simulink model "stateflow_test"  (R2021a)
settings: Solver=FixedStepAuto  StartTime=0.0  StopTime=10.0  FixedStep=1/64  RelTol=1e-3
settings Model: OrderedModelArguments=off  Creator=Jack-STK2  LastModifiedBy=jacky

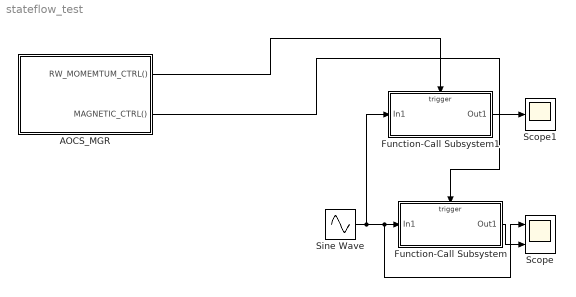
== system stateflow_test ==
  AOCS_MGR : Stateflow chart  TreatAsAtomicUnit=on  SystemSampleTime=1/8
  Function-Call Subsystem : Subsystem  TreatAsAtomicUnit=on
  Function-Call Subsystem1 : Subsystem  TreatAsAtomicUnit=on
  Scope : Scope  NumInputPorts=2
  Scope1 : Scope
  Sine Wave : Sin  Frequency=2*pi  SampleTime=0
  wires:
  Sine Wave/1 -> Function-Call Subsystem1/1(In1), Scope/1, Function-Call Subsystem/1(In1)
  Function-Call Subsystem/1(Out1) -> Scope/2
  AOCS_MGR/2(MAGNETIC_CTRL()) -> Function-Call Subsystem/Trigger
  AOCS_MGR/1(RW_MOMEMTUM_CTRL()) -> Function-Call Subsystem1/Trigger
  Function-Call Subsystem1/1(Out1) -> Scope1/1

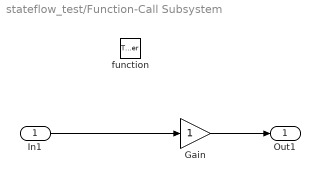
== system stateflow_test/Function-Call Subsystem ==
  In1 : Inport
  function : TriggerPort  TriggerType=function-call  VariantControl=(inherit)
  Gain : Gain
  Out1 : Outport
  wires:
  In1/1 -> Gain/1
  Gain/1 -> Out1/1

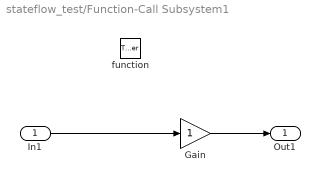
== system stateflow_test/Function-Call Subsystem1 ==
  In1 : Inport
  function : TriggerPort  TriggerType=function-call  VariantControl=(inherit)
  Gain : Gain
  Out1 : Outport
  wires:
  Gain/1 -> Out1/1
  In1/1 -> Gain/1

== stateflow chart stateflow_test/AOCS_MGR ==
  state ASH_CTRL [parallel]
    du:
    if ~in(ASH_CTRL.OFF)
    RW_MOMEMTUM_CTRL
    end
    settings: executionOrder=2
    state OFF
    state MTQ_ONLY
      entry, during:
      MAGNETIC_CTRL
    state MTQ_AND_RW
    (default) -> OFF
    OFF -> MTQ_ONLY : SCHEDULE_OBJECT
    MTQ_ONLY -> MTQ_AND_RW : SELECT_MTQ_AND_RW
    MTQ_AND_RW -> MTQ_ONLY : SELECT_MTQ_ONLY
  state ASH [parallel]
    settings: executionOrder=1
    state IDLE
    state STABILIZE
      entry, during:
      stabilize_processing;
    state SLO
    state STRA
    (default) -> IDLE
    IDLE -> STABILIZE : [C1]{A1}
    SLO -> STABILIZE
    STABILIZE -> STRA : [C2]{A2}
    STRA -> SLO : [C3]
  data: object_state local Enum: ASHMODE size=1; C function_output boolean size=1; C function_output; C function_output; fsw parameter; count_stab local double size=1; count_day_night local double size=1
  events: SELECT_MTQ_AND_RW local FUNCTION_CALL_EVENT; SELECT_MTQ_ONLY local FUNCTION_CALL_EVENT; SCHEDULE_OBJECT local FUNCTION_CALL_EVENT; RW_MOMEMTUM_CTRL output FUNCTION_CALL_EVENT; MAGNETIC_CTRL output FUNCTION_CALL_EVENT
  function A1:
    | function A1
    | % global ash_mgr_object_state
    | % disp(objet_state)
    | % disp(objet_state *2);%'STABILIZE';
    | count_stab = 0;
    | send(ASH_CTRL.SCHEDULE_OBJECT, ASH_CTRL.OFF);
    | % send(ASH_CTRL.SCHEDULE_OBJECT);
    | 
    | % send(ASH_CTRL.SCHEDULE_OBJECT);
    | 
    | ASH.object_state = ASHMODE.STAB;
    | % ash_mgr_object_state = ASHMODE.STAB;
  function C = C1:
    | function C = C1
    | % Check that all necessary equipments for the STABILIZE submode are ON
    | C = true;
  function C = C2:
    | function C = C2
    | C = true;%stablized;
  function A2:
    | function A2
    | % global ash_mgr_object_state
    | % disp(objet_state)
    | % disp(objet_state *2);%'STABILIZE';
    | %  ash_mgr_object_state = ASHMODE.STRA;
    |  send(ASH_CTRL.SCHEDULE_OBJECT, ASH_CTRL.MTQ_ONLY);
    | ASH.object_state = ASHMODE.STRA;
    | count_day_night = 0;
  function stabilize_processing:
    | function stabilize_processing
    | if  0 < fsw.ash_mgr.epsilon
    |     count_stab = count_stab+1;
    | else
    |     count_stab = 0;
    | end
  function C = C3:
    | function C = C3
    | C = count_day_night >= fsw.ash_mgr.Tconf;
  function A3:
    | function A3
    | % global ash_mgr_object_state
    | % disp(objet_state)
    | % disp(objet_state *2);%'STABILIZE';
    | %  ash_mgr_object_state = ASHMODE.STRA;
    | send(ASH_CTRL.SELECT_MTQ_AND_RW, ASH_CTRL.MTQ_AND_RW);
    | ASH.object_state = ASHMODE.STRA;
